simulink model "MotorSpeedSimulinkControl"  (R2015b)
settings: Solver=VariableStepAuto  StartTime=0.0  StopTime=10.0  RelTol=1e-3
values from neighbouring files (symbols this model uses):
  b = str2num(get(handles.frictionText,'String'))    [MotorSpeedSimulinkModeling.m]
  J = str2num(get(handles.inertiaText,'String'))    [MotorSpeedSimulinkModeling.m]
  Ke = str2num(get(handles.emfText,'String'))    [MotorSpeedSimulinkModeling.m]
  Kt = str2num(get(handles.torqueText,'String'))    [MotorSpeedSimulinkModeling.m]
  L = str2num(get(handles.inductionText,'String'))    [MotorSpeedSimulinkModeling.m]
  R = str2num(get(handles.resistanceText,'String'))    [MotorSpeedSimulinkModeling.m]
libraries: simulink x1
settings Model: Creator=YOUNG  LastModifiedBy=YOUNG

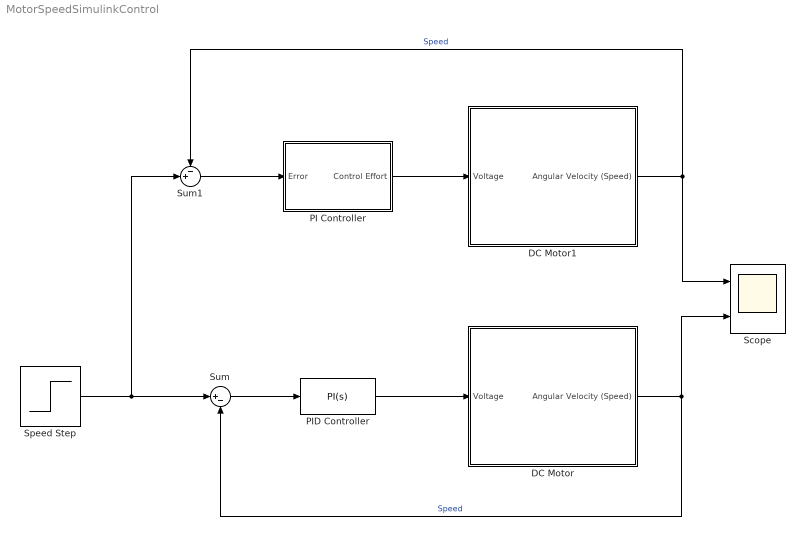
== system MotorSpeedSimulinkControl ==
  DC Motor : Subsystem
      mask Display: image(imread('dc_motor_diagram.png'));
  DC Motor1 : Subsystem
      mask Display: image(imread('dc_motor_diagram.png'));
  PI Controller : Subsystem
  PID Controller : simulink/Continuous/PID Controller  Controller=PI  TimeDomain=Continuous-time  SampleTime=-1  IntegratorMethod=Forward Euler  FilterMethod=Forward Euler  Form=Parallel  UseFilter=on  ControllerParametersSource=internal  P=19.0989843060353  I=35.8793652986903  D=2.63394762562422  N=559.738561067247  InitialConditionSource=internal  InitialConditionForIntegrator=0  InitialConditionForFilter=0  ExternalReset=none  LimitOutput=off  UpperSaturationLimit=inf  LowerSaturationLimit=-inf  LinearizeAsGain=on  AntiWindupMode=none  Kb=1  TrackingMode=off  Kt=1  PParamMin=[]  PParamMax=[]  IParamMin=[]  IParamMax=[]  DParamMin=[]  DParamMax=[]  NParamMin=[]  NParamMax=[]  KbParamMin=[]  KbParamMax=[]  KtParamMin=[]  KtParamMax=[]  POutMin=[]  POutMax=[]  IOutMin=[]  IOutMax=[]  DOutMin=[]  DOutMax=[]  NOutMin=[]  NOutMax=[]  KbOutMin=[]  KbOutMax=[]  KtOutMin=[]  KtOutMax=[]  IntegratorOutMin=[]  IntegratorOutMax=[]  FilterOutMin=[]  FilterOutMax=[]  SumOutMin=[]  SumOutMax=[]  SumI1OutMin=[]  SumI1OutMax=[]  SumI2OutMin=[]  SumI2OutMax=[]  SumI3OutMin=[]  SumI3OutMax=[]  SumDOutMin=[]  SumDOutMax=[]  SaturationOutMin=[]  SaturationOutMax=[]  IntegratorContinuousStateAttributes=''  IntegratorStateMustResolveToSignalObject=off  IntegratorRTWStateStorageClass=Auto  FilterContinuousStateAttributes=''  FilterStateMustResolveToSignalObject=off  FilterRTWStateStorageClass=Auto  DifferentiatorICPrevScaledInput=0  DifferentiatorOutMin=[]  DifferentiatorOutMax=[]
  Scope : Scope  NumInputPorts=2
  Speed Step : Step  Time=0  SampleTime=0
  Sum : Sum  Inputs=|+-
  Sum1 : Sum  Inputs=-+|
  wires:
  PID Controller/1 -> DC Motor/1(Voltage)
  DC Motor/1(Angular Velocity (Speed)) -> Scope/2, Sum/2  "Speed"
  Speed Step/1 -> Sum1/2, Sum/1
  Sum/1 -> PID Controller/1
  DC Motor1/1(Angular Velocity (Speed)) -> Scope/1, Sum1/1  "Speed"
  Sum1/1 -> PI Controller/1(Error)
  PI Controller/1(Control Effort) -> DC Motor1/1(Voltage)

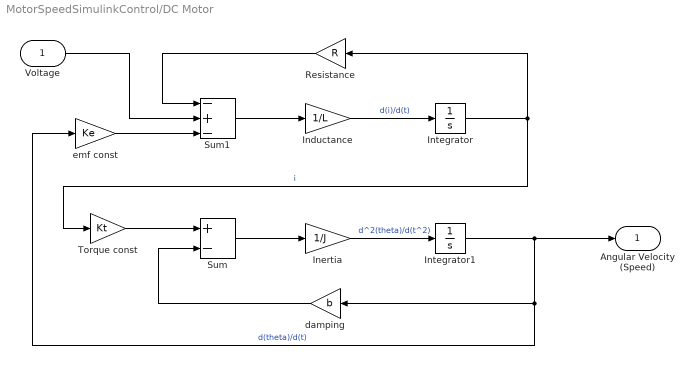
== system MotorSpeedSimulinkControl/DC Motor ==
  Voltage : Inport
  Inductance : Gain  Gain=1/L
  Inertia : Gain  Gain=1/J
  Integrator : Integrator
  Integrator1 : Integrator
  Resistance : Gain  Gain=R
  Sum : Sum  Inputs=+-
  Sum1 : Sum  Inputs=-+-
  Torque const : Gain  Gain=Kt
  damping : Gain  Gain=b
  emf const : Gain  Gain=Ke
  Angular Velocity (Speed) : Outport
  wires:
  damping/1 -> Sum/2
  Resistance/1 -> Sum1/1
  Inductance/1 -> Integrator/1  "d(i)/d(t)"
  Integrator/1 -> Torque const/1, Resistance/1  "i"
  emf const/1 -> Sum1/3
  Voltage/1 -> Sum1/2
  Sum/1 -> Inertia/1
  Torque const/1 -> Sum/1
  Sum1/1 -> Inductance/1
  Inertia/1 -> Integrator1/1  "d^2(theta)/d(t^2)"
  Integrator1/1 -> Angular Velocity (Speed)/1, damping/1, emf const/1  "d(theta)/d(t)"

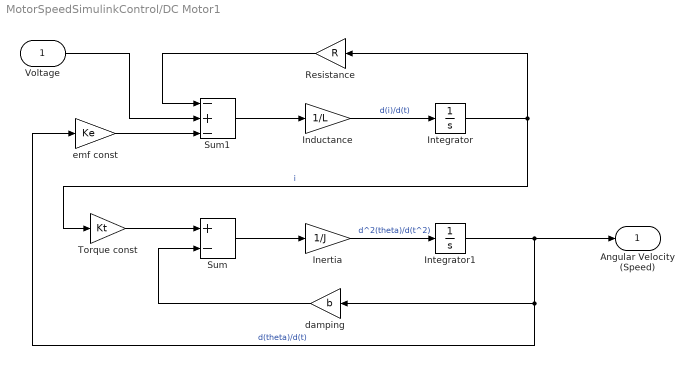
== system MotorSpeedSimulinkControl/DC Motor1 ==
  Voltage : Inport
  Inductance : Gain  Gain=1/L
  Inertia : Gain  Gain=1/J
  Integrator : Integrator
  Integrator1 : Integrator
  Resistance : Gain  Gain=R
  Sum : Sum  Inputs=+-
  Sum1 : Sum  Inputs=-+-
  Torque const : Gain  Gain=Kt
  damping : Gain  Gain=b
  emf const : Gain  Gain=Ke
  Angular Velocity (Speed) : Outport
  wires:
  damping/1 -> Sum/2
  Resistance/1 -> Sum1/1
  Inductance/1 -> Integrator/1  "d(i)/d(t)"
  Integrator/1 -> Torque const/1, Resistance/1  "i"
  emf const/1 -> Sum1/3
  Voltage/1 -> Sum1/2
  Sum/1 -> Inertia/1
  Torque const/1 -> Sum/1
  Sum1/1 -> Inductance/1
  Inertia/1 -> Integrator1/1  "d^2(theta)/d(t^2)"
  Integrator1/1 -> Angular Velocity (Speed)/1, damping/1, emf const/1  "d(theta)/d(t)"

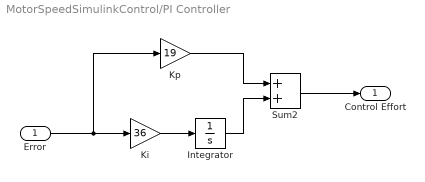
== system MotorSpeedSimulinkControl/PI Controller ==
  Error : Inport
  Integrator : Integrator
  Ki : Gain  Gain=36
  Kp : Gain  Gain=19
  Sum2 : Sum
  Control Effort : Outport
  wires:
  Error/1 -> Kp/1, Ki/1
  Sum2/1 -> Control Effort/1
  Integrator/1 -> Sum2/2
  Ki/1 -> Integrator/1
  Kp/1 -> Sum2/1
